simulink model "Power_Factor_Correction_Final_Simulation"  (R2024a)
settings: Solver=VariableStepAuto  StartTime=0.0  StopTime=10  RelTol=1e-3
libraries: spsSeriesRLCBranchLib x17, spsBreakerLib x16, spsRMSLib x7, simulink x2, eePowerMeasurement x2, dspsigops x2, spsVoltageMeasurementLib x2, spsACVoltageSourceLib x1, spsCurrentMeasurementLib x1, embmathops x1, spsSeriesRLCLoadLib x1, sps_lib x1
settings Model: Creator=DELL  LastModifiedBy=DELL

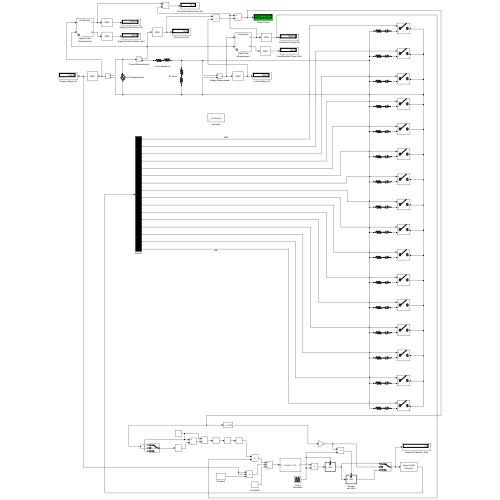
[thumbnail: Simulink's stored preview of the top-level diagram]
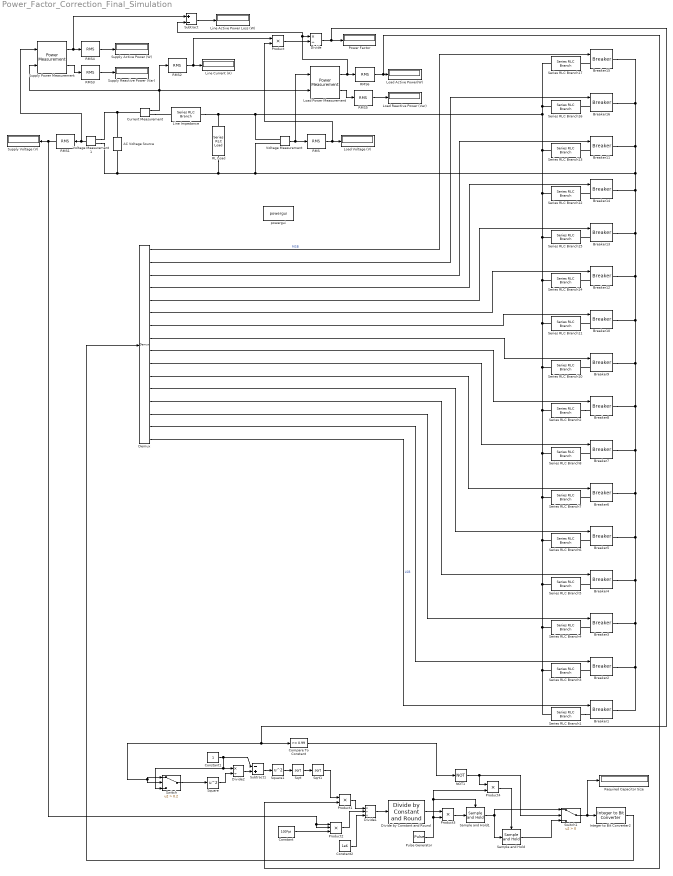
== system Power_Factor_Correction_Final_Simulation ==
  AC Voltage Source : spsACVoltageSourceLib/AC Voltage Source  Amplitude=230*sqrt(2)  Phase=0  Frequency=50  SampleTime=0  Measurements=None  BusType=swing  Pref=10e3  Qref=0  Qmin=-inf  Qmax=+inf
  Breaker{1..16} (16 alike) : spsBreakerLib/Breaker  InitialState=0  SwitchingTimes="[1/60  5/60]"  External=on  BreakerResistance=0  SnubberResistance=0  SnubberCapacitance=0  Measurements=None  MoreParameters=on  NoBreakLoop=off
  Compare To Constant : simulink/Logic and Bit Operations/Compare To Constant  relop=>=  const=0.99  OutDataTypeStr=boolean
  Constant : Constant  Value=100*pi
  Constant1 : Constant
  Constant2 : Constant  Value=1e6
  Current Measurement : spsCurrentMeasurementLib/Current Measurement  PhasorSimulation=off  OutputType=Complex  PSBequivalent=0
  Demux : Demux  Outputs=16
  Divide : Product  Inputs=*/  RndMeth=Zero  SaturateOnIntegerOverflow=on
  Divide by Constant and Round : embmathops/Divide by Constant and Round  Denominator=1  RoundingMethod=Floor  SimulateUsing=Code generation
      settings: LibrarySourceBlock=embeddedMathLib/Divide by Constant and Round
  Divide1 : Product  Inputs=*/*
  Divide2 : Product  Inputs=*/
  Integer to Bit Converter2 : simulink/Logic and Bit Operations/Integer to Bit Converter  nbits=16  signedInputValues=Unsigned  bitOrder=MSB first  outDtype=Inherit via internal rule
  Line Active Power Loss (W) : Display
  Line Current (A) : Display
      settings: Format=bank
  Line Impedance : spsSeriesRLCBranchLib/Series RLC Branch  LConnTagsString=__new0  RConnTagsString=__new0  BranchType=RL  Resistance=0.1  Inductance=1e-3  SetiL0=off  InitialCurrent=0  Capacitance=0  Setx0=off  InitialVoltage=0  Measurements=None
  Load Active Power(W) : Display
      settings: Format=bank
  Load Power Measurement : eePowerMeasurement/Power Measurement  LabelModeActiveChoice=Continuous  F=50  K=[1]  Ts=0
  Load Reactive Power (Var) : Display
      settings: Format=bank
  Load Voltage (V) : Display
      settings: Format=bank
  NOT1 : Logic  Operator=NOT  IconShape=distinctive  AllPortsSameDT=off  OutDataTypeStr=boolean
  Power Factor : Display
  Product{,1,3..4} (4 alike) : Product
  Product2 : Product  Inputs=3
  Pulse Generator : DiscretePulseGenerator  PulseType=Time based  Period=0.5  PulseWidth=0.1  PhaseDelay=0.5
  RL Load : spsSeriesRLCLoadLib/Series RLC Load  LConnTagsString=a  RConnTagsString=__new0  NominalVoltage=230  NominalFrequency=50  ActivePower=3000  InductivePower=3000  CapacitivePower=0  Setx0=off  InitialVoltage=0  SetiL0=off  InitialCurrent=0  Measurements=None  LoadType=constant Z
  RMS{,1..6} (7 alike) : spsRMSLib/RMS  TrueRMS=on  Freq=50  RMSInit=230  Ts=0
  Required Capacitor Size : Display
  Sample and Hold : dspsigops/Sample and Hold  trig=Rising edge  initCond=0  latchinput=off
  Sample and Hold1 : dspsigops/Sample and Hold  trig=Rising edge  initCond=0  latchinput=off
  Series RLC Branch1 : spsSeriesRLCBranchLib/Series RLC Branch  LConnTagsString=__new0  RConnTagsString=__new0  BranchType=RC  Resistance=0.00001  Inductance=1e-3  SetiL0=off  InitialCurrent=0  Capacitance=1e-6  Setx0=off  InitialVoltage=0  Measurements=None
  Series RLC Branch10 : spsSeriesRLCBranchLib/Series RLC Branch  LConnTagsString=__new0  RConnTagsString=__new0  BranchType=RC  Resistance=0.00001  Inductance=1e-3  SetiL0=off  InitialCurrent=0  Capacitance=256e-6  Setx0=off  InitialVoltage=0  Measurements=None
  Series RLC Branch11 : spsSeriesRLCBranchLib/Series RLC Branch  LConnTagsString=__new0  RConnTagsString=__new0  BranchType=RC  Resistance=0.00001  Inductance=1e-3  SetiL0=off  InitialCurrent=0  Capacitance=512e-6  Setx0=off  InitialVoltage=0  Measurements=None
  Series RLC Branch12 : spsSeriesRLCBranchLib/Series RLC Branch  LConnTagsString=__new0  RConnTagsString=__new0  BranchType=RC  Resistance=0.00001  Inductance=1e-3  SetiL0=off  InitialCurrent=0  Capacitance=4096e-6  Setx0=off  InitialVoltage=0  Measurements=None
  Series RLC Branch13 : spsSeriesRLCBranchLib/Series RLC Branch  LConnTagsString=__new0  RConnTagsString=__new0  BranchType=RC  Resistance=0.00001  Inductance=1e-3  SetiL0=off  InitialCurrent=0  Capacitance=8192e-6  Setx0=off  InitialVoltage=0  Measurements=None
  Series RLC Branch14 : spsSeriesRLCBranchLib/Series RLC Branch  LConnTagsString=__new0  RConnTagsString=__new0  BranchType=RC  Resistance=0.00001  Inductance=1e-3  SetiL0=off  InitialCurrent=0  Capacitance=1024e-6  Setx0=off  InitialVoltage=0  Measurements=None
  Series RLC Branch15 : spsSeriesRLCBranchLib/Series RLC Branch  LConnTagsString=__new0  RConnTagsString=__new0  BranchType=RC  Resistance=0.00001  Inductance=1e-3  SetiL0=off  InitialCurrent=0  Capacitance=2048e-6  Setx0=off  InitialVoltage=0  Measurements=None
  Series RLC Branch16 : spsSeriesRLCBranchLib/Series RLC Branch  LConnTagsString=__new0  RConnTagsString=__new0  BranchType=RC  Resistance=0.00001  Inductance=1e-3  SetiL0=off  InitialCurrent=0  Capacitance=16384e-6  Setx0=off  InitialVoltage=0  Measurements=None
  Series RLC Branch17 : spsSeriesRLCBranchLib/Series RLC Branch  LConnTagsString=__new0  RConnTagsString=__new0  BranchType=RC  Resistance=0.00001  Inductance=1e-3  SetiL0=off  InitialCurrent=0  Capacitance=32768e-6  Setx0=off  InitialVoltage=0  Measurements=None
  Series RLC Branch2 : spsSeriesRLCBranchLib/Series RLC Branch  LConnTagsString=__new0  RConnTagsString=__new0  BranchType=RC  Resistance=0.00001  Inductance=1e-3  SetiL0=off  InitialCurrent=0  Capacitance=128e-6  Setx0=off  InitialVoltage=0  Measurements=None
  Series RLC Branch3 : spsSeriesRLCBranchLib/Series RLC Branch  LConnTagsString=__new0  RConnTagsString=__new0  BranchType=RC  Resistance=0.00001  Inductance=1e-3  SetiL0=off  InitialCurrent=0  Capacitance=2e-6  Setx0=off  InitialVoltage=0  Measurements=None
  Series RLC Branch4 : spsSeriesRLCBranchLib/Series RLC Branch  LConnTagsString=__new0  RConnTagsString=__new0  BranchType=RC  Resistance=0.00001  Inductance=1e-3  SetiL0=off  InitialCurrent=0  Capacitance=4e-6  Setx0=off  InitialVoltage=0  Measurements=None
  Series RLC Branch5 : spsSeriesRLCBranchLib/Series RLC Branch  LConnTagsString=__new0  RConnTagsString=__new0  BranchType=RC  Resistance=0.00001  Inductance=1e-3  SetiL0=off  InitialCurrent=0  Capacitance=8e-6  Setx0=off  InitialVoltage=0  Measurements=None
  Series RLC Branch6 : spsSeriesRLCBranchLib/Series RLC Branch  LConnTagsString=__new0  RConnTagsString=__new0  BranchType=RC  Resistance=0.00001  Inductance=1e-3  SetiL0=off  InitialCurrent=0  Capacitance=16e-6  Setx0=off  InitialVoltage=0  Measurements=None
  Series RLC Branch7 : spsSeriesRLCBranchLib/Series RLC Branch  LConnTagsString=__new0  RConnTagsString=__new0  BranchType=RC  Resistance=0.00001  Inductance=1e-3  SetiL0=off  InitialCurrent=0  Capacitance=32e-6  Setx0=off  InitialVoltage=0  Measurements=None
  Series RLC Branch8 : spsSeriesRLCBranchLib/Series RLC Branch  LConnTagsString=__new0  RConnTagsString=__new0  BranchType=RC  Resistance=0.00001  Inductance=1e-3  SetiL0=off  InitialCurrent=0  Capacitance=64e-6  Setx0=off  InitialVoltage=0  Measurements=None
  Sqrt : Sqrt
  Sqrt1 : Sqrt
  Square : Math  Operator=square
  Square1 : Math  Operator=square
  Subtract : Sum  Inputs=+-
  Subtract1 : Sum  Inputs=-+
  Supply Active Power (W) : Display
      settings: Format=bank  Decimation=3
  Supply Power Measurement : eePowerMeasurement/Power Measurement  LabelModeActiveChoice=Continuous  F=50  K=[1]  Ts=0
  Supply Reactive Power (Var) : Display
      settings: Format=bank
  Supply Voltage (V) : Display
      settings: Format=bank
  Switch : Switch  Criteria=u2 > Threshold  Threshold=0.2  SaturateOnIntegerOverflow=off  InputSameDT=off
  Switch1 : Switch  Criteria=u2 > Threshold  SaturateOnIntegerOverflow=off  InputSameDT=off
  Voltage Measurement : spsVoltageMeasurementLib/Voltage Measurement  PhasorSimulation=off  OutputType=Complex  PSBequivalent=0
  Voltage Measurement1 : spsVoltageMeasurementLib/Voltage Measurement  PhasorSimulation=off  OutputType=Complex  PSBequivalent=0
  powergui : sps_lib/powergui  Priority=1  SimulationMode=Continuous  SampleTime=50e-6  frequency=60  Iterations=50  frequencyindice=50  Pbase=100e6  ErrMax=1e-4  UnitsV=kV  UnitsW=MW  buscounter=0  FunctionMessages=off  echomessages=off  EnableUseOfTLC=off  CurrentSourceSwitches=off  DisableSnubberDevices=off  DisableRonSwitches=off  DisableVfSwitches=off  DisplayEquations=off  AutomaticDiscreteSolvers=off  SolverType=Tustin/Backward Euler (TBE)  Interpol=off  ExternalGateDelay=off  methode=off  Ts=100  x0status=blocks  SPID=on  SwTol=0  HookPort=off  NonlinearTolerance=1e-4  nMaxIteration=100  ContinueOnMaxIteration=off  RestoreLinks=warning  ResistiveCurrentMeasurement=off  Frange=[0:2:500]  Ylog=off  Xlog=on  ShowGrid=off  save=off  variable=ZData  structure=0  ZoomFFT=off  StartTime=0.0  cycles=1  DisplayStyle=1  fundamental=60  FreqAxis=off  MaxFrequency=1000  frequencyindicesteady=1  RmsSteady=1  display=off
  wires:
  Voltage Measurement/1 -> Load Power Measurement/1, RMS/1
  RMS/1 -> Product/2, Load Voltage (V)/1
  Voltage Measurement1/1 -> Supply Power Measurement/1, RMS1/1
  RMS1/1 -> Supply Voltage (V)/1, Product2/2, Product2/1
  RMS2/1 -> Product/1, Line Current (A)/1
  Current Measurement/1 -> Supply Power Measurement/2, RMS2/1, Load Power Measurement/2
  RMS3/1 -> Supply Reactive Power (Var)/1
  RMS4/1 -> Supply Active Power (W)/1
  Supply Power Measurement/1 -> Subtract/1, RMS4/1
  Supply Power Measurement/2 -> RMS3/1
  RMS5/1 -> Load Reactive Power (Var)/1
  Load Power Measurement/2 -> RMS5/1
  RMS6/1 -> Load Active Power(W)/1, Product1/2
  Load Power Measurement/1 -> Subtract/2, Divide/1, RMS6/1
  Product/1 -> Divide/2
  Divide/1 -> Power Factor/1, Compare To Constant/1, Switch/1, Switch/2
  Subtract/1 -> Line Active Power Loss (W)/1
  Compare To Constant/1 -> NOT1/1
  Integer to Bit Converter2/1 -> Demux/1
  Demux/16 -> Breaker1/1  "LSB"
  Demux/15 -> Breaker2/1
  Demux/14 -> Breaker3/1
  Demux/13 -> Breaker4/1
  Demux/12 -> Breaker5/1
  Demux/11 -> Breaker6/1
  Demux/10 -> Breaker7/1
  Demux/9 -> Breaker8/1
  Demux/8 -> Breaker9/1
  Demux/7 -> Breaker10/1
  Demux/6 -> Breaker12/1
  Demux/5 -> Breaker13/1
  Demux/4 -> Breaker14/1
  Demux/3 -> Breaker11/1
  Demux/2 -> Breaker16/1
  Demux/1 -> Breaker15/1  "MSB"
  Product1/1 -> Divide1/1
  Constant/1 -> Product2/3
  Product2/1 -> Divide1/2
  Constant1/1 -> Switch/3, Divide2/1, Subtract1/1
  Square/1 -> Divide2/2
  Divide2/1 -> Subtract1/2
  Subtract1/1 -> Square1/1
  Sqrt/1 -> Sqrt1/1
  Divide1/1 -> Divide by Constant and Round/1
  Constant2/1 -> Divide1/3
  Switch/1 -> Square/1
  Pulse Generator/1 -> Product3/2, Sample and Hold1/Trigger, Product4/2
  Divide by Constant and Round/1 -> Product3/1
  Product3/1 -> Sample and Hold1/1
  Sample and Hold1/1 -> Switch1/1, Sample and Hold/1
  Switch1/1 -> Required Capacitor Size/1, Integer to Bit Converter2/1
  NOT1/1 -> Product4/1, Switch1/2
  Sample and Hold/1 -> Switch1/3
  Product4/1 -> Sample and Hold/Trigger
  Sqrt1/1 -> Product1/1
  Square1/1 -> Sqrt/1
  connections:
  AC Voltage Source/RConn1 -- Voltage Measurement1/LConn1 -- Current Measurement/LConn1
  Current Measurement/RConn1 -- Line Impedance/LConn1
  Voltage Measurement/LConn2 -- Breaker11/RConn1 -- Breaker15/RConn1 -- Breaker16/RConn1 -- Breaker14/RConn1 -- Breaker13/RConn1 -- Breaker10/RConn1 -- Breaker9/RConn1 -- Breaker8/RConn1 -- Breaker7/RConn1 -- Breaker6/RConn1 -- Breaker5/RConn1 -- Breaker4/RConn1 -- Breaker3/RConn1 -- Breaker2/RConn1 -- Breaker1/RConn1 -- Breaker12/RConn1 -- RL Load/RConn1 -- Voltage Measurement1/LConn2 -- AC Voltage Source/LConn1
  Series RLC Branch1/RConn1 -- Breaker1/LConn1
  Breaker2/LConn1 -- Series RLC Branch3/RConn1
  Breaker3/LConn1 -- Series RLC Branch4/RConn1
  Breaker4/LConn1 -- Series RLC Branch5/RConn1
  Breaker5/LConn1 -- Series RLC Branch6/RConn1
  Breaker7/LConn1 -- Series RLC Branch8/RConn1
  Breaker6/LConn1 -- Series RLC Branch7/RConn1
  Breaker9/LConn1 -- Series RLC Branch10/RConn1
  Breaker10/LConn1 -- Series RLC Branch11/RConn1
  Series RLC Branch2/RConn1 -- Breaker8/LConn1
  Breaker14/LConn1 -- Series RLC Branch12/RConn1
  Breaker11/LConn1 -- Series RLC Branch13/RConn1
  Breaker13/LConn1 -- Series RLC Branch15/RConn1
  Breaker12/LConn1 -- Series RLC Branch14/RConn1
  Series RLC Branch1/LConn1 -- Series RLC Branch3/LConn1 -- Series RLC Branch4/LConn1 -- Series RLC Branch5/LConn1 -- Series RLC Branch6/LConn1 -- Series RLC Branch13/LConn1 -- Series RLC Branch17/LConn1 -- Series RLC Branch16/LConn1 -- Voltage Measurement/LConn1 -- Line Impedance/RConn1 -- RL Load/LConn1 -- Series RLC Branch12/LConn1 -- Series RLC Branch15/LConn1 -- Series RLC Branch14/LConn1 -- Series RLC Branch11/LConn1 -- Series RLC Branch10/LConn1 -- Series RLC Branch2/LConn1 -- Series RLC Branch8/LConn1 -- Series RLC Branch7/LConn1
  Breaker16/LConn1 -- Series RLC Branch16/RConn1
  Breaker15/LConn1 -- Series RLC Branch17/RConn1
